simulink model "buck_boost_l1"  (R2023a)
settings: Solver=FixedStepAuto  StartTime=0.0  StopTime=0.3  FixedStep=ts  RelTol=1e-3
values from neighbouring files (symbols this model uses):
  C = 330e-6    (= 0.00033)    [init.m]
  fsw = 10e3    (= 10000)    [init.m]
  ki = 20    [init.m]
  kp = 0    [init.m]
  L = 100e-6    (= 0.0001)    [init.m]
  R = 5    [init.m]
  ts = 1e-6    (= 1e-06)    [init.m]
  vin = 100    [init.m]
libraries: simulink x2
settings Model: Creator=ptrujillo  LastModifiedBy=pablo
settings SolverCC: AlgebraicLoopSolver=TrustRegion
settings DataIOCC: ReturnWorkspaceOutputs=off
settings DebuggingCC: UnconnectedInputMsg=warning  UnconnectedOutputMsg=warning  UnconnectedLineMsg=warning  ArithmeticOperatorsInVariantConditions=warning
settings ModelReferenceCC: EnableRefExpFcnMdlSchedulingChecks=on
settings SFSimCC: CustomCodeUndefinedFunction=UseInterfaceOnly

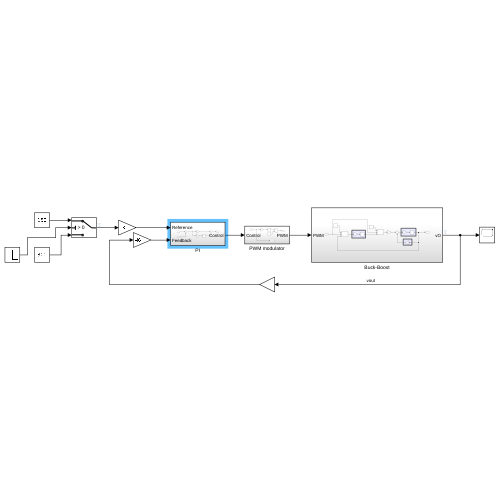
[thumbnail: Simulink's stored preview of the top-level diagram]
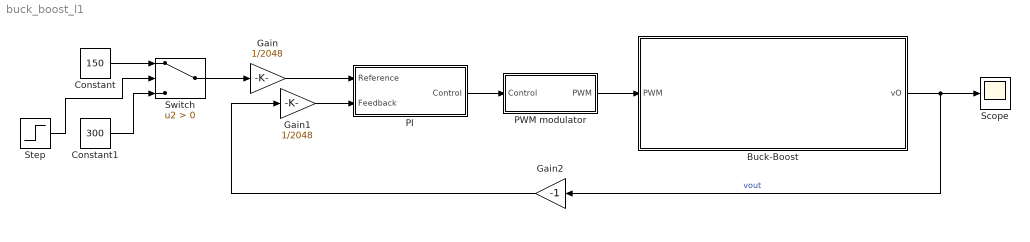
== system buck_boost_l1 ==
  Buck-Boost : Subsystem
  Constant : Constant  Value=150
  Constant1 : Constant  Value=300
  Gain : Gain  Gain=1/2048
  Gain1 : Gain  Gain=1/2048
  Gain2 : Gain  Gain=-1
  PI : Subsystem
  PWM modulator : Subsystem
  Scope : Scope
  Step : Step  Time=0.15  Before=1  After=0  SampleTime=0
  Switch : Switch  Criteria=u2 > Threshold  SaturateOnIntegerOverflow=off  InputSameDT=off
  wires:
  Buck-Boost/1(vO) -> Gain2/1, Scope/1  "vout"
  Gain2/1 -> Gain1/1
  PI/1(Control) -> PWM modulator/1(Control)
  PWM modulator/1(PWM) -> Buck-Boost/1("PWM ")
  Constant/1 -> Switch/1
  Switch/1 -> Gain/1
  Constant1/1 -> Switch/3
  Step/1 -> Switch/2
  Gain/1 -> PI/1(Reference)
  Gain1/1 -> PI/2(Feedback)

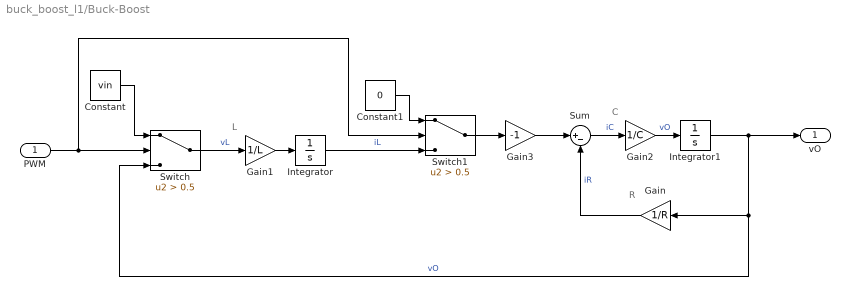
== system buck_boost_l1/Buck-Boost ==
  note: R
  note: C
  note: L
  "PWM " : Inport
  Constant : Constant  Value=vin
  Constant1 : Constant  Value=0
  Gain : Gain  Gain=1/R
  Gain1 : Gain  Gain=1/L
  Gain2 : Gain  Gain=1/C
  Gain3 : Gain  Gain=-1
  Integrator : Integrator
  Integrator1 : Integrator
  Sum : Sum  Inputs=|+-
  Switch : Switch  Criteria=u2 > Threshold  Threshold=0.5  SaturateOnIntegerOverflow=off  InputSameDT=off
  Switch1 : Switch  Criteria=u2 > Threshold  Threshold=0.5  SaturateOnIntegerOverflow=off  InputSameDT=off
  vO : Outport  VectorParamsAs1DForOutWhenUnconnected=off
  wires:
  Constant1/1 -> Switch1/1
  Integrator/1 -> Switch1/3  "iL"
  "PWM "/1 -> Switch1/2, Switch/2
  Sum/1 -> Gain2/1  "iC"
  Constant/1 -> Switch/1
  Switch1/1 -> Gain3/1
  Integrator1/1 -> vO/1, Switch/3, Gain/1  "vO"
  Gain/1 -> Sum/2  "iR"
  Switch/1 -> Gain1/1  "vL"
  Gain1/1 -> Integrator/1
  Gain2/1 -> Integrator1/1  "vO"
  Gain3/1 -> Sum/1

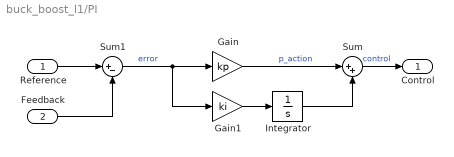
== system buck_boost_l1/PI ==
  Reference : Inport
  Feedback : Inport  Port=2
  Gain : Gain  Gain=kp
  Gain1 : Gain  Gain=ki
  Integrator : Integrator
  Sum : Sum  Inputs=|++
  Sum1 : Sum  Inputs=|+-
  Control : Outport  VectorParamsAs1DForOutWhenUnconnected=off
  wires:
  Gain1/1 -> Integrator/1
  Integrator/1 -> Sum/2
  Feedback/1 -> Sum1/2
  Sum1/1 -> Gain1/1, Gain/1  "error"
  Reference/1 -> Sum1/1
  Gain/1 -> Sum/1  "p_action"
  Sum/1 -> Control/1  "control"

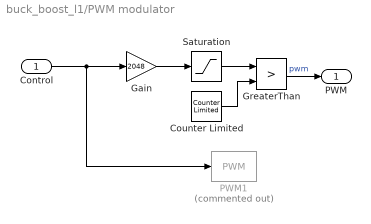
== system buck_boost_l1/PWM modulator ==
  Control : Inport
  Counter Limited : simulink/Sources/Counter Limited  uplimit=100  tsamp=-1
  Gain : Gain  Gain=2048
  GreaterThan : RelationalOperator  Operator=>  OutDataTypeStr=boolean  RndMeth=Simplest  InputSameDT=off
  PWM1 : simulink/Discontinuities/PWM  Commented=on  DisableCoverage=on  Period=1/fsw  InitialDelay=0  DisallowZeroDutyCycle=off  RunAtFixedTimeIntervals=on  SampleTime=ts
  Saturation : Saturate  UpperLimit=90  LowerLimit=0
  PWM : Outport  VectorParamsAs1DForOutWhenUnconnected=off
  wires:
  Saturation/1 -> GreaterThan/1
  Counter Limited/1 -> GreaterThan/2
  Control/1 -> PWM1/1, Gain/1
  GreaterThan/1 -> PWM/1  "pwm"
  Gain/1 -> Saturation/1
